simulink model "bloques_P"  (R2021b)
settings: Solver=FixedStepAuto  StartTime=0.0  StopTime=Tc  FixedStep=Ts  RelTol=1e-3
values from neighbouring files (symbols this model uses):
  a = 210.90461*(Ts*Ts)    (= 2.1090461e-06)    [raiz.m]
  b = 25.65696*Ts - 2.0    (= -1.997434304)    [raiz.m]
  c = 1.0 - 25.65696*Ts + 210.90461*(Ts*Ts)    (= 0.997436413046)    [raiz.m]
  e = 2.14036*Ts*Ts    (= 2.14036e-08)    [raiz.m]
  Kp = 3    [raiz.m]
  sp = 0.0    (= 0)    [raiz.m]
  Tz = 0.002    [raiz.m]
settings Model: Creator=yeezvs  LastModifiedBy=yeezvs
settings DataIOCC: ReturnWorkspaceOutputs=off

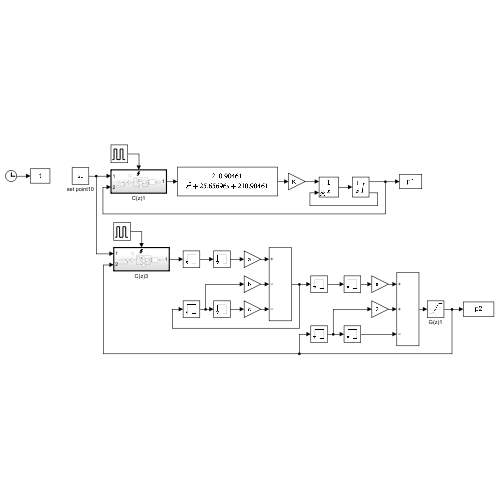
[thumbnail: Simulink's stored preview of the top-level diagram]
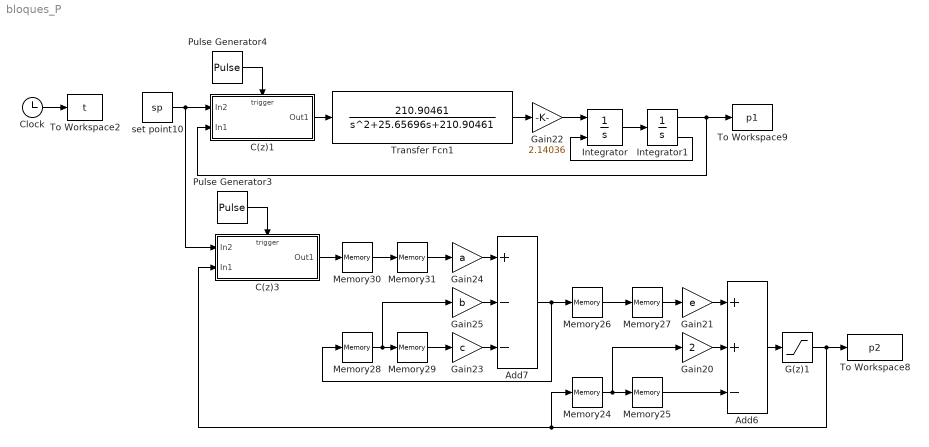
== system bloques_P ==
  Add6 : Sum  Inputs=++-
  Add7 : Sum  Inputs=+--
  C(z)1 : Subsystem  TreatAsAtomicUnit=on
  C(z)3 : Subsystem  TreatAsAtomicUnit=on
  Clock : Clock
  G(z)1 : Saturate  UpperLimit=0.15  LowerLimit=-0.15
  Gain20 : Gain  Gain=2
  Gain21 : Gain  Gain=e
  Gain22 : Gain  Gain=2.14036
  Gain23 : Gain  Gain=c
  Gain24 : Gain  Gain=a
  Gain25 : Gain  Gain=b
  Integrator : Integrator  ExternalReset=either
  Integrator1 : Integrator  InitialCondition=-0.15  LimitOutput=on  UpperSaturationLimit=0.15  LowerSaturationLimit=-0.15  ShowSaturationPort=on
  Memory24 : Memory  InitialCondition=-0.15
  Memory25 : Memory  InitialCondition=-0.15
  Memory{26..31} (6 alike) : Memory
  Pulse Generator3 : DiscretePulseGenerator  PulseType=Time based  Period=Tz  PulseWidth=50
  Pulse Generator4 : DiscretePulseGenerator  PulseType=Time based  Period=Tz  PulseWidth=50
  To Workspace2 : ToWorkspace  VariableName=t  SampleTime=-1
      settings: Save2DSignal=2-D array (concatenate along first dimension)
  To Workspace8 : ToWorkspace  VariableName=p2  SampleTime=-1
      settings: Save2DSignal=2-D array (concatenate along first dimension)
  To Workspace9 : ToWorkspace  VariableName=p1  SampleTime=-1
      settings: Save2DSignal=2-D array (concatenate along first dimension)
  Transfer Fcn1 : TransferFcn  Numerator=[210.90461]  Denominator=[1 25.65696 210.90461]
  set point10 : Constant  Value=sp
  wires:
  Clock/1 -> To Workspace2/1
  Memory31/1 -> Gain24/1
  Add7/1 -> Memory26/1, Memory28/1
  Memory29/1 -> Gain23/1
  Gain23/1 -> Add7/3
  Gain20/1 -> Add6/2
  Add6/1 -> G(z)1/1
  Memory26/1 -> Memory27/1
  Memory27/1 -> Gain21/1
  Memory25/1 -> Add6/3
  Gain24/1 -> Add7/1
  Gain25/1 -> Add7/2
  Memory30/1 -> Memory31/1
  Gain21/1 -> Add6/1
  Memory28/1 -> Gain25/1, Memory29/1
  C(z)3/1(Out1) -> Memory30/1
  Pulse Generator3/1 -> C(z)3/Trigger
  G(z)1/1 -> To Workspace8/1, C(z)3/2(In1), Memory24/1
  Memory24/1 -> Memory25/1, Gain20/1
  set point10/1 -> C(z)1/1(In2), C(z)3/1(In2)
  Pulse Generator4/1 -> C(z)1/Trigger
  C(z)1/1(Out1) -> Transfer Fcn1/1
  Transfer Fcn1/1 -> Gain22/1
  Integrator/1 -> Integrator1/1
  Integrator1/2 -> Integrator/2
  Gain22/1 -> Integrator/1
  Integrator1/1 -> C(z)1/2(In1), To Workspace9/1

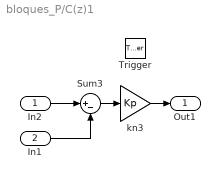
== system bloques_P/C(z)1 ==
  In2 : Inport
  In1 : Inport  Port=2
  Trigger : TriggerPort  VariantControl=(inherit)
  Sum3 : Sum  Inputs=|+-
  kn3 : Gain  Gain=Kp
  Out1 : Outport
  wires:
  In2/1 -> Sum3/1
  Sum3/1 -> kn3/1
  In1/1 -> Sum3/2
  kn3/1 -> Out1/1

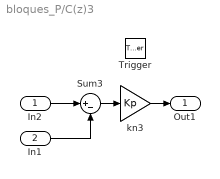
== system bloques_P/C(z)3 ==
  In2 : Inport
  In1 : Inport  Port=2
  Trigger : TriggerPort  VariantControl=(inherit)
  Sum3 : Sum  Inputs=|+-
  kn3 : Gain  Gain=Kp
  Out1 : Outport
  wires:
  In2/1 -> Sum3/1
  Sum3/1 -> kn3/1
  In1/1 -> Sum3/2
  kn3/1 -> Out1/1
